simulink model "untitled1"  (R2020b)
settings: Solver=VariableStepAuto  StartTime=0.0  StopTime=10.0  RelTol=1e-3
model workspace (MAT data in the model file):
  f = -1
undefined symbols (not defined in the file or in its folder): duration, effort, index, joint_name, left_wheel_hinge, model_name, pioneer2dx, right_wheel_hinge, sampleTime, waypoints
libraries: robotgazebolib x13, simulink x4, robotcorelib x3, robotalgslib x1
settings Model: Creator=tfpeng  LastModifiedBy=tfpeng

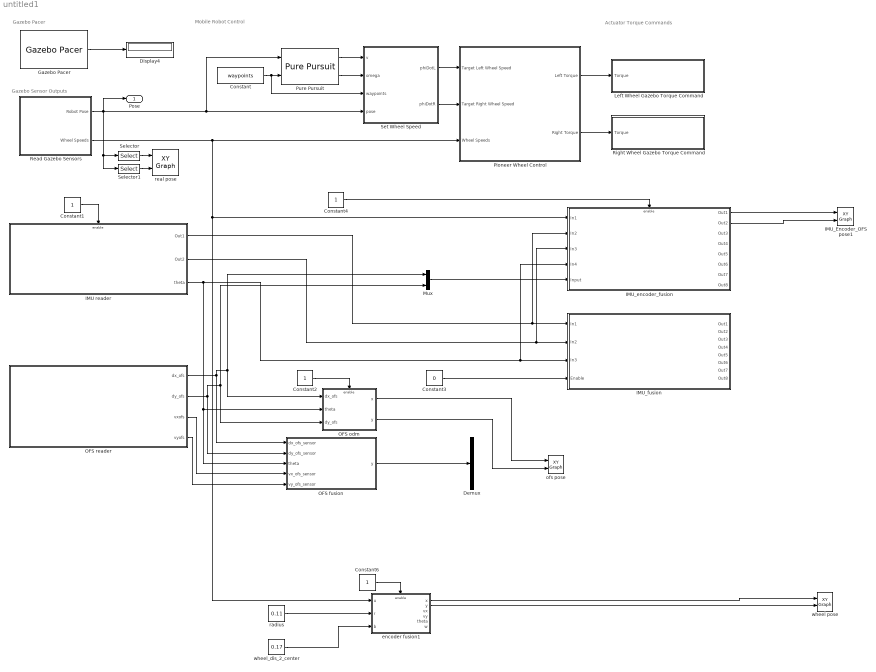
== system untitled1 ==
  note: Gazebo Pacer
  note: Actuator Torque Commands
  note: Mobile Robot Control
  note: Gazebo Sensor Outputs
  Constant : Constant  Value=waypoints
  Constant{1..2,4,6} (4 alike) : Constant
  Constant3 : Constant  Value=0
  Demux : Demux  Outputs=8
  Display4 : Display
  Gazebo Pacer : robotgazebolib/Gazebo Pacer  ResetBehavior=Reset Gazebo simulation time and scene  SampleTime=0.01
      settings: SourceProductName=Robotics System Toolbox
  IMU reader : Subsystem
  IMU_Encoder_OFS pose1 : simulink/Sinks/XY Graph  xmin=-1  xmax=4  ymin=-1  ymax=8  st=-1
  IMU_encoder_fusion : Subsystem
  IMU_fusion : Subsystem
  Left Wheel Gazebo Torque Command : Subsystem
  Mux : Mux  Inputs=2
  OFS fusion : MATLAB Function  TreatAsAtomicUnit=on
  OFS odm : Subsystem
  OFS reader : Subsystem
  Pioneer Wheel Control : Subsystem
  Pure Pursuit : robotalgslib/Pure Pursuit  DesiredLinearVelocity=1.0  MaxAngularVelocity=1.0  LookaheadDistance=1.0  TargetDirPort=off  SimulateUsing=Code generation
  Read Gazebo Sensors : Subsystem
  Right Wheel Gazebo Torque Command : Subsystem
  Selector : Selector  InputPortWidth=3  IndexOptions=Index vector (dialog)  Indices=[1]  OutputSizes=1
  Selector1 : Selector  InputPortWidth=3  IndexOptions=Index vector (dialog)  Indices=[2]  OutputSizes=1
  Set Wheel Speed : MATLAB Function  TreatAsAtomicUnit=on
  encoder fusion1 : Subsystem  TreatAsAtomicUnit=on
  ofs pose : simulink/Sinks/XY Graph  xmin=-1  xmax=4  ymin=-1  ymax=8  st=-1
  radius : Constant  Value=0.11
  real pose : simulink/Sinks/XY Graph  xmin=-1  xmax=4  ymin=-1  ymax=8  st=-1
  wheel pose : simulink/Sinks/XY Graph  xmin=-1  xmax=4  ymin=-1  ymax=8  st=-1
  wheel_dis_2_center : Constant  Value=0.17
  Pose : Outport
  wires:
  Pure Pursuit/2 -> Set Wheel Speed/2(omega)
  Constant/1 -> Set Wheel Speed/3(waypoints), Pure Pursuit/2
  Pioneer Wheel Control/2(Right Torque) -> Right Wheel Gazebo Torque Command/1(Torque)
  Pure Pursuit/1 -> Set Wheel Speed/1(v)
  Read Gazebo Sensors/1(Robot Pose) -> Selector1/1, Selector/1, Pure Pursuit/1, Set Wheel Speed/4(pose), Pose/1
  Set Wheel Speed/2(phiDotR) -> Pioneer Wheel Control/2(Target Right Wheel Speed)
  Set Wheel Speed/1(phiDotL) -> Pioneer Wheel Control/1(Target Left Wheel Speed)
  Pioneer Wheel Control/1(Left Torque) -> Left Wheel Gazebo Torque Command/1(Torque)
  Gazebo Pacer/1 -> Display4/1
  Read Gazebo Sensors/2(Wheel Speeds) -> encoder fusion1/1(u), IMU_encoder_fusion/1(In1), Pioneer Wheel Control/3(Wheel Speeds)
  radius/1 -> encoder fusion1/2(r)
  wheel_dis_2_center/1 -> encoder fusion1/3(b)
  Selector/1 -> real pose/1
  Selector1/1 -> real pose/2
  Constant4/1 -> IMU_encoder_fusion/Enable
  Constant6/1 -> encoder fusion1/Enable
  encoder fusion1/1(x) -> wheel pose/1
  encoder fusion1/2(y) -> wheel pose/2
  IMU reader/1(Out1) -> IMU_encoder_fusion/2(In2), IMU_fusion/1(In1)
  IMU reader/2(Out2) -> IMU_encoder_fusion/3(In3), IMU_fusion/2(In2)
  Constant3/1 -> IMU_fusion/4(Enable)
  Constant1/1 -> IMU reader/Enable
  IMU_encoder_fusion/1(Out1) -> IMU_Encoder_OFS pose1/1
  IMU_encoder_fusion/2(Out2) -> IMU_Encoder_OFS pose1/2
  OFS reader/1(dx_ofs) -> OFS odm/1(dx_ofs), Mux/1, OFS fusion/1(dx_ofs_sensor)
  OFS reader/2(dy_ofs) -> OFS odm/3(dy_ofs), Mux/2, OFS fusion/2(dy_ofs_sensor)
  Mux/1 -> IMU_encoder_fusion/5(Input)
  IMU reader/3(theta) -> OFS fusion/3(theta), OFS odm/2(theta), IMU_encoder_fusion/4(In4), IMU_fusion/3(In3)
  Constant2/1 -> OFS odm/Enable
  OFS reader/3(vxofs) -> OFS fusion/4(vx_ofs_sensor)
  OFS reader/4(vyofs) -> OFS fusion/5(vy_ofs_sensor)
  OFS fusion/1(y) -> Demux/1
  OFS odm/1(x) -> ofs pose/1
  OFS odm/2(y) -> ofs pose/2

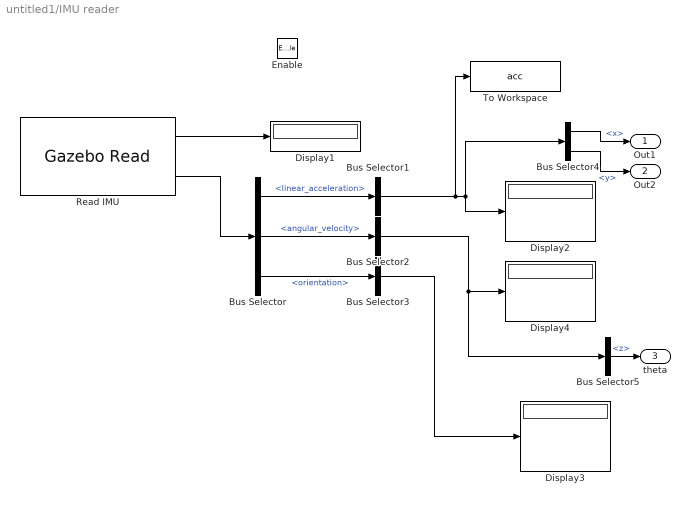
== system untitled1/IMU reader ==
  Enable : EnablePort
  Bus Selector : BusSelector  OutputSignals=linear_acceleration,angular_velocity,orientation
  Bus Selector1 : BusSelector  OutputSignals=x,y,z  OutputAsBus=on
  Bus Selector2 : BusSelector  OutputSignals=x,y,z  OutputAsBus=on
  Bus Selector3 : BusSelector  OutputSignals=w,x,y,z  OutputAsBus=on
  Bus Selector4 : BusSelector  OutputSignals=x,y
  Bus Selector5 : BusSelector  OutputSignals=z
  Display{1..4} (4 alike) : Display
      Display2 settings: Decimation=3
      Display3 settings: Decimation=3
      Display4 settings: Decimation=3
  Read IMU : robotgazebolib/Gazebo Read  topicSource=From Gazebo  topic=/gazebo/default/pioneer2dx/imu/imu/imu  messageType=gazebo_msgs/IMU  sampleTime=0.01
      settings: SourceProductName=Robotics System Toolbox
  To Workspace : ToWorkspace  VariableName=acc  SaveFormat=Timeseries  SampleTime=-1
      settings: Decimation=3
  Out1 : Outport
  Out2 : Outport  Port=2
  theta : Outport  Port=3
  wires:
  Bus Selector2/1 -> Bus Selector5/1, Display4/1
  Read IMU/1 -> Display1/1
  Read IMU/2 -> Bus Selector/1
  Bus Selector3/1 -> Display3/1
  Bus Selector/3 -> Bus Selector3/1  "<orientation>"
  Bus Selector/1 -> Bus Selector1/1  "<linear_acceleration>"
  Bus Selector1/1 -> To Workspace/1, Display2/1, Bus Selector4/1
  Bus Selector/2 -> Bus Selector2/1  "<angular_velocity>"
  Bus Selector4/1 -> Out1/1  "<x>"
  Bus Selector4/2 -> Out2/1  "<y>"
  Bus Selector5/1 -> theta/1  "<z>"

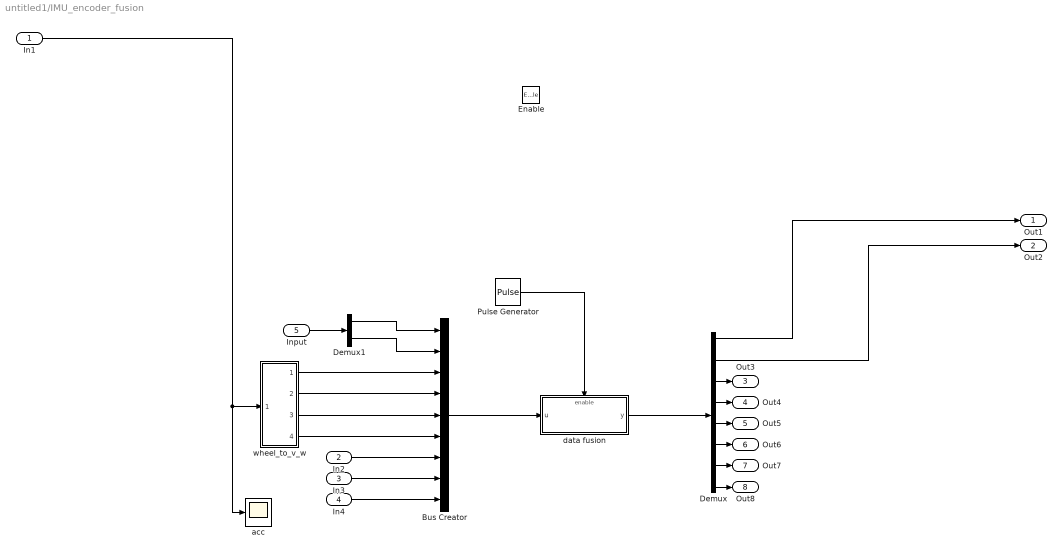
== system untitled1/IMU_encoder_fusion ==
  In1 : Inport
  In2 : Inport  Port=2
  In3 : Inport  Port=3
  In4 : Inport  Port=4
  Input : Inport  Port=5
  Enable : EnablePort
  Bus Creator : BusCreator  Inputs=9
  Demux : Demux  Outputs=8
  Demux1 : Demux  Outputs=2
  Pulse Generator : DiscretePulseGenerator  PulseType=Time based  Period=0.01  PulseWidth=50
  acc : Scope
  data fusion : Subsystem  TreatAsAtomicUnit=on
  wheel_to_v_w : Subsystem
  Out1 : Outport
  Out2 : Outport  Port=2
  Out3 : Outport  Port=3
  Out4 : Outport  Port=4
  Out5 : Outport  Port=5
  Out6 : Outport  Port=6
  Out7 : Outport  Port=7
  Out8 : Outport  Port=8
  wires:
  wheel_to_v_w/1(Out1) -> Bus Creator/3
  Demux/7 -> Out7/1
  Demux/8 -> Out8/1
  Pulse Generator/1 -> data fusion/Enable
  Demux/2 -> Out2/1
  In2/1 -> Bus Creator/7
  Demux/3 -> Out3/1
  In4/1 -> Bus Creator/9
  In1/1 -> acc/1, wheel_to_v_w/1(In1)
  In3/1 -> Bus Creator/8
  data fusion/1(y) -> Demux/1
  Demux/4 -> Out4/1
  Demux/1 -> Out1/1
  Demux/5 -> Out5/1
  Bus Creator/1 -> data fusion/1(u)
  Demux/6 -> Out6/1
  wheel_to_v_w/3(Out4) -> Bus Creator/5
  wheel_to_v_w/2(Out3) -> Bus Creator/4
  wheel_to_v_w/4(Out2) -> Bus Creator/6
  Input/1 -> Demux1/1
  Demux1/1 -> Bus Creator/1
  Demux1/2 -> Bus Creator/2

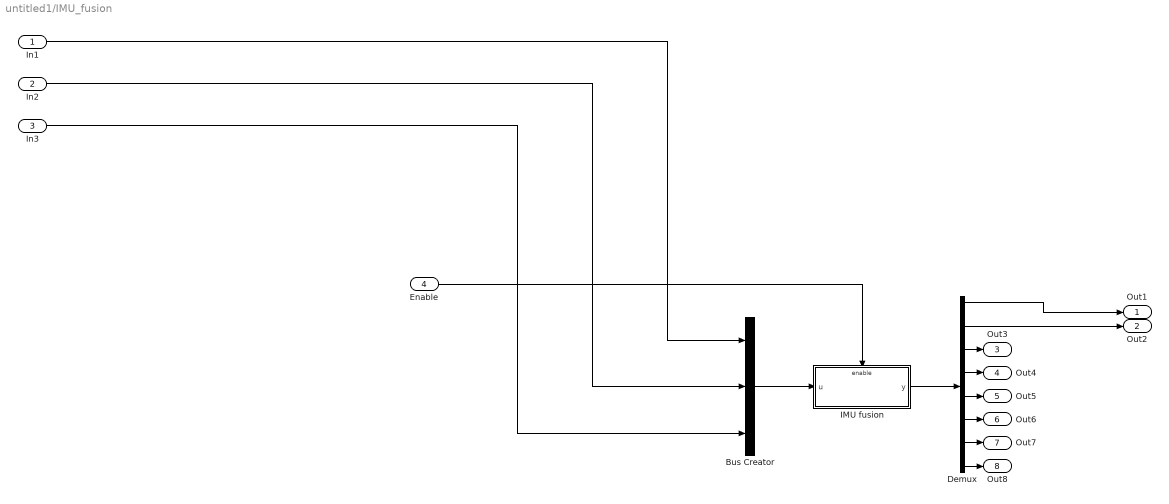
== system untitled1/IMU_fusion ==
  In1 : Inport
  In2 : Inport  Port=2
  In3 : Inport  Port=3
  Enable : Inport  Port=4
  Bus Creator : BusCreator  Inputs=3
  Demux : Demux  Outputs=8
  IMU fusion : Subsystem  TreatAsAtomicUnit=on
  Out1 : Outport
  Out2 : Outport  Port=2
  Out3 : Outport  Port=3
  Out4 : Outport  Port=4
  Out5 : Outport  Port=5
  Out6 : Outport  Port=6
  Out7 : Outport  Port=7
  Out8 : Outport  Port=8
  wires:
  Demux/3 -> Out3/1
  Enable/1 -> IMU fusion/Enable
  Demux/5 -> Out5/1
  Bus Creator/1 -> IMU fusion/1(u)
  In3/1 -> Bus Creator/3
  Demux/4 -> Out4/1
  IMU fusion/1(y) -> Demux/1
  Demux/6 -> Out6/1
  In2/1 -> Bus Creator/2
  In1/1 -> Bus Creator/1
  Demux/7 -> Out7/1
  Demux/2 -> Out2/1
  Demux/8 -> Out8/1
  Demux/1 -> Out1/1

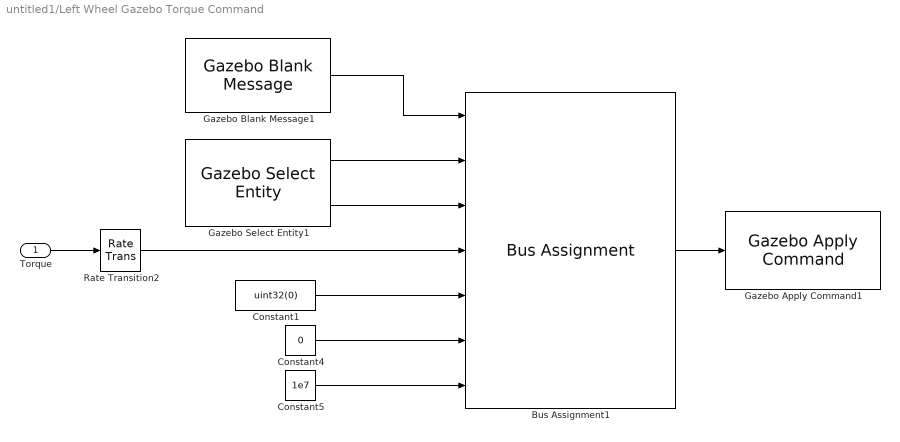
== system untitled1/Left Wheel Gazebo Torque Command ==
  Torque : Inport
  Bus Assignment1 : BusAssignment  AssignedSignals=model_name,joint_name,effort,index,duration.seconds,duration.nano_seconds
  Constant1 : Constant  Value=uint32(0)
  Constant4 : Constant  Value=0
  Constant5 : Constant  Value=1e7
  Gazebo Apply Command1 : robotgazebolib/Gazebo Apply Command  cmdType=ApplyJointTorque  sampleTime=0.01
      settings: SourceProductName=Robotics System Toolbox
  Gazebo Blank Message1 : robotgazebolib/Gazebo Blank Message  msgType=ApplyJointTorque  sampleTime=0.01  busName='Gazebo_SL_Bus_gazebo_msgs_ApplyJointTorque'
      settings: SourceProductName=Robotics System Toolbox
  Gazebo Select Entity1 : robotgazebolib/Gazebo Select Entity  modelElemName=pioneer2dx/left_wheel_hinge  outputArraySize=128  OutputLabel=Joint  SelectType=Joint
      settings: SourceProductName=Robotics System Toolbox
  Rate Transition2 : RateTransition
  wires:
  Bus Assignment1/1 -> Gazebo Apply Command1/1
  Constant5/1 -> Bus Assignment1/7
  Gazebo Blank Message1/1 -> Bus Assignment1/1
  Gazebo Select Entity1/2 -> Bus Assignment1/3
  Gazebo Select Entity1/1 -> Bus Assignment1/2
  Torque/1 -> Rate Transition2/1
  Constant4/1 -> Bus Assignment1/6
  Rate Transition2/1 -> Bus Assignment1/4
  Constant1/1 -> Bus Assignment1/5

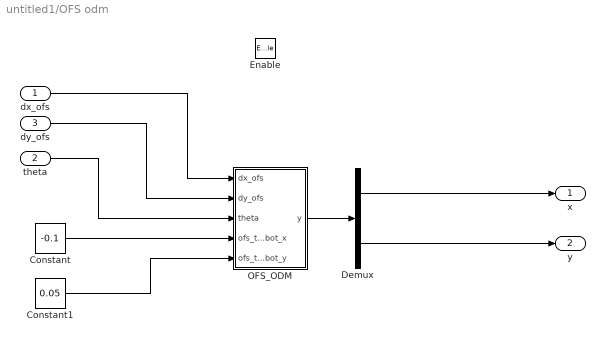
== system untitled1/OFS odm ==
  dx_ofs : Inport
  theta : Inport  Port=2
  dy_ofs : Inport  Port=3
  Enable : EnablePort
  Constant : Constant  Value=-0.1
  Constant1 : Constant  Value=0.05
  Demux : Demux  Outputs=2
  OFS_ODM : MATLAB Function  TreatAsAtomicUnit=on
  x : Outport
  y : Outport  Port=2
  wires:
  Demux/2 -> y/1
  Demux/1 -> x/1
  theta/1 -> OFS_ODM/3(theta)
  dx_ofs/1 -> OFS_ODM/1(dx_ofs)
  OFS_ODM/1(y) -> Demux/1
  dy_ofs/1 -> OFS_ODM/2(dy_ofs)
  Constant/1 -> OFS_ODM/4(ofs_to_robot_x)
  Constant1/1 -> OFS_ODM/5(ofs_to_robot_y)

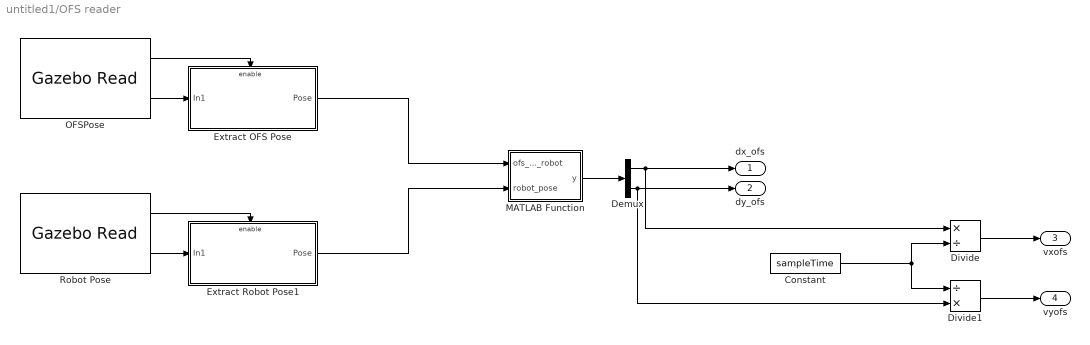
== system untitled1/OFS reader ==
  Constant : Constant  Value=sampleTime
  Demux : Demux  Outputs=2
  Divide : Product  Inputs=*/
  Divide1 : Product  Inputs=/*
  Extract OFS Pose : Subsystem
  Extract Robot Pose1 : Subsystem
  MATLAB Function : MATLAB Function  TreatAsAtomicUnit=on
  OFSPose : robotgazebolib/Gazebo Read  topicSource=From Gazebo  topic=/gazebo/ground_truth/link_state/pioneer2dx/ofs  messageType=gazebo_msgs/LinkState  sampleTime=0.01
      settings: SourceProductName=Robotics System Toolbox
  Robot Pose : robotgazebolib/Gazebo Read  topicSource=From Gazebo  topic=/gazebo/ground_truth/world_pose/pioneer2dx/chassis  messageType=gazebo_msgs/Pose  sampleTime=0.01
      settings: SourceProductName=Robotics System Toolbox
  dx_ofs : Outport
  dy_ofs : Outport  Port=2
  vxofs : Outport  Port=3
  vyofs : Outport  Port=4
  wires:
  Extract Robot Pose1/1(Pose) -> MATLAB Function/2(robot_pose)
  Extract OFS Pose/1(Pose) -> MATLAB Function/1(ofs_pose_robot)
  MATLAB Function/1(y) -> Demux/1
  Robot Pose/1 -> Extract Robot Pose1/Enable
  OFSPose/1 -> Extract OFS Pose/Enable
  Robot Pose/2 -> Extract Robot Pose1/1(In1)
  OFSPose/2 -> Extract OFS Pose/1(In1)
  Demux/1 -> dx_ofs/1, Divide/1
  Demux/2 -> Divide1/2, dy_ofs/1
  Constant/1 -> Divide/2, Divide1/1
  Divide/1 -> vxofs/1
  Divide1/1 -> vyofs/1

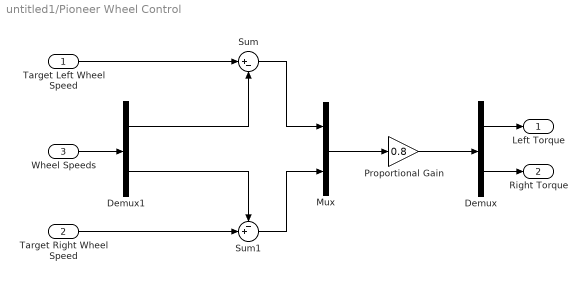
== system untitled1/Pioneer Wheel Control ==
  Target Left Wheel Speed : Inport
  Target Right Wheel Speed : Inport  Port=2
  Wheel Speeds : Inport  Port=3
  Demux : Demux  Outputs=2
  Demux1 : Demux  Outputs=2
  Mux : Mux  Inputs=2
  Proportional Gain : Gain  Gain=0.8
  Sum : Sum  Inputs=|+-
  Sum1 : Sum  Inputs=-+|
  Left Torque : Outport
  Right Torque : Outport  Port=2
  wires:
  Sum1/1 -> Mux/2
  Target Left Wheel Speed/1 -> Sum/1
  Sum/1 -> Mux/1
  Mux/1 -> Proportional Gain/1
  Proportional Gain/1 -> Demux/1
  Demux/1 -> Left Torque/1
  Demux/2 -> Right Torque/1
  Wheel Speeds/1 -> Demux1/1
  Demux1/1 -> Sum/2
  Target Right Wheel Speed/1 -> Sum1/2
  Demux1/2 -> Sum1/1

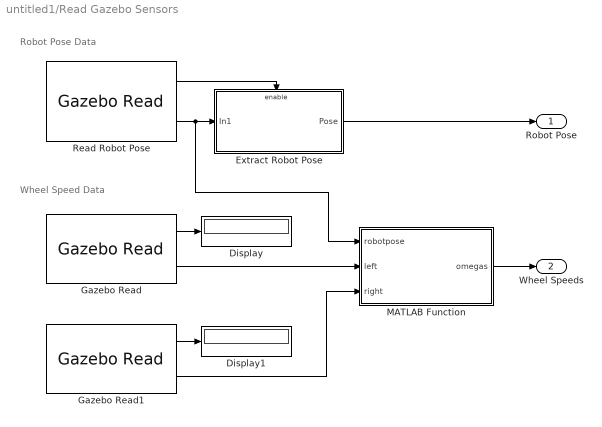
== system untitled1/Read Gazebo Sensors ==
  note: Robot Pose Data
  note: Wheel Speed Data
  Display : Display
  Display1 : Display
  Extract Robot Pose : Subsystem
  Gazebo Read : robotgazebolib/Gazebo Read  topicSource=From Gazebo  topic=/gazebo/ground_truth/world_pose/pioneer2dx/left_wheel  messageType=gazebo_msgs/Pose  sampleTime=0.01
      settings: SourceProductName=Robotics System Toolbox
  Gazebo Read1 : robotgazebolib/Gazebo Read  topicSource=From Gazebo  topic=/gazebo/ground_truth/world_pose/pioneer2dx/right_wheel  messageType=gazebo_msgs/Pose  sampleTime=0.01
      settings: SourceProductName=Robotics System Toolbox
  MATLAB Function : MATLAB Function  TreatAsAtomicUnit=on
  Read Robot Pose : robotgazebolib/Gazebo Read  topicSource=From Gazebo  topic=/gazebo/ground_truth/world_pose/pioneer2dx/chassis  messageType=gazebo_msgs/Pose  sampleTime=0.01
      settings: SourceProductName=Robotics System Toolbox
  Robot Pose : Outport
  Wheel Speeds : Outport  Port=2
  wires:
  Read Robot Pose/2 -> MATLAB Function/1(robotpose), Extract Robot Pose/1(In1)
  Extract Robot Pose/1(Pose) -> Robot Pose/1
  Read Robot Pose/1 -> Extract Robot Pose/Enable
  Gazebo Read/1 -> Display/1
  Gazebo Read1/1 -> Display1/1
  MATLAB Function/1(omegas) -> Wheel Speeds/1
  Gazebo Read/2 -> MATLAB Function/2(left)
  Gazebo Read1/2 -> MATLAB Function/3(right)

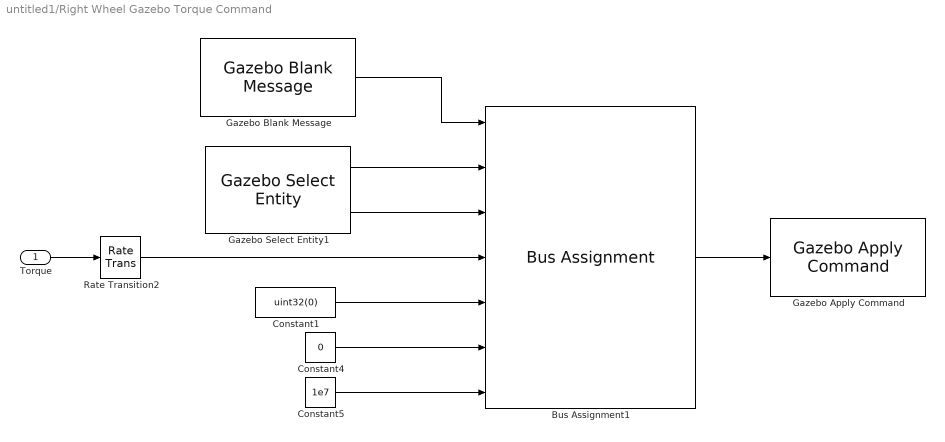
== system untitled1/Right Wheel Gazebo Torque Command ==
  Torque : Inport
  Bus Assignment1 : BusAssignment  AssignedSignals=model_name,joint_name,effort,index,duration.seconds,duration.nano_seconds
  Constant1 : Constant  Value=uint32(0)
  Constant4 : Constant  Value=0
  Constant5 : Constant  Value=1e7
  Gazebo Apply Command : robotgazebolib/Gazebo Apply Command  cmdType=ApplyJointTorque  sampleTime=0.01
      settings: SourceProductName=Robotics System Toolbox
  Gazebo Blank Message : robotgazebolib/Gazebo Blank Message  msgType=ApplyJointTorque  sampleTime=0.01  busName='Gazebo_SL_Bus_gazebo_msgs_ApplyJointTorque'
      settings: SourceProductName=Robotics System Toolbox
  Gazebo Select Entity1 : robotgazebolib/Gazebo Select Entity  modelElemName=pioneer2dx/right_wheel_hinge  outputArraySize=128  OutputLabel=Joint  SelectType=Joint
      settings: SourceProductName=Robotics System Toolbox
  Rate Transition2 : RateTransition
  wires:
  Constant1/1 -> Bus Assignment1/5
  Rate Transition2/1 -> Bus Assignment1/4
  Constant4/1 -> Bus Assignment1/6
  Torque/1 -> Rate Transition2/1
  Gazebo Select Entity1/1 -> Bus Assignment1/2
  Gazebo Select Entity1/2 -> Bus Assignment1/3
  Gazebo Blank Message/1 -> Bus Assignment1/1
  Constant5/1 -> Bus Assignment1/7
  Bus Assignment1/1 -> Gazebo Apply Command/1

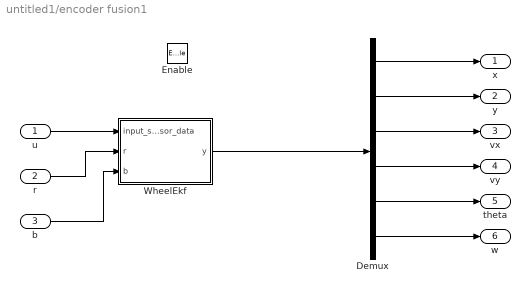
== system untitled1/encoder fusion1 ==
  u : Inport
  r : Inport  Port=2
  b : Inport  Port=3
  Enable : EnablePort
  Demux : Demux  Outputs=6
  WheelEkf : MATLAB Function  TreatAsAtomicUnit=on
  x : Outport
  y : Outport  Port=2
  vx : Outport  Port=3
  vy : Outport  Port=4
  theta : Outport  Port=5
  w : Outport  Port=6
  wires:
  u/1 -> WheelEkf/1(input_sensor_data)
  WheelEkf/1(y) -> Demux/1
  r/1 -> WheelEkf/2(r)
  b/1 -> WheelEkf/3(b)
  Demux/1 -> x/1
  Demux/2 -> y/1
  Demux/3 -> vx/1
  Demux/4 -> vy/1
  Demux/5 -> theta/1
  Demux/6 -> w/1

== system untitled1/IMU_encoder_fusion/data fusion ==
  u : Inport
  Enable : EnablePort
  PoseEstimationEkf : MATLAB Function  TreatAsAtomicUnit=on
  y : Outport
  wires:
  u/1 -> PoseEstimationEkf/1(input_sensor_data)
  PoseEstimationEkf/1(y) -> y/1

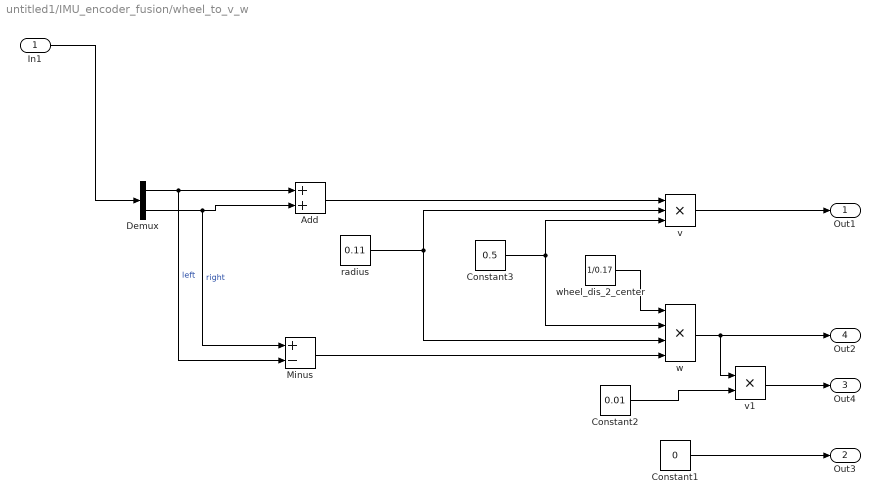
== system untitled1/IMU_encoder_fusion/wheel_to_v_w ==
  In1 : Inport
  Add : Sum
  Constant1 : Constant  Value=0
  Constant2 : Constant  Value=0.01
  Constant3 : Constant  Value=0.5
  Demux : Demux  Outputs=2
  Minus : Sum  Inputs=+-
  radius : Constant  Value=0.11
  v : Product  Inputs=3
  v1 : Product
  w : Product  Inputs=4
  wheel_dis_2_center : Constant  Value=1/0.17
  Out1 : Outport
  Out3 : Outport  Port=2
  Out4 : Outport  Port=3
  Out2 : Outport  Port=4
  wires:
  Minus/1 -> w/4
  w/1 -> v1/1, Out2/1
  In1/1 -> Demux/1
  Add/1 -> v/1
  wheel_dis_2_center/1 -> w/1
  v/1 -> Out1/1
  radius/1 -> w/3, v/2
  Demux/2 -> Minus/1, Add/2  "right"
  Demux/1 -> Minus/2, Add/1  "left"
  Constant3/1 -> w/2, v/3
  Constant1/1 -> Out3/1
  Constant2/1 -> v1/2
  v1/1 -> Out4/1

== system untitled1/IMU_fusion/IMU fusion ==
  u : Inport
  Enable : EnablePort
  PoseEstimationEkf : MATLAB Function  TreatAsAtomicUnit=on
  y : Outport
  wires:
  u/1 -> PoseEstimationEkf/1(input_sensor_data)
  PoseEstimationEkf/1(y) -> y/1

== system untitled1/OFS reader/Extract OFS Pose ==
  note: Generate a pose vector (x, y, theta) from X, Y, and quaternion data
  In1 : Inport
  Enable : EnablePort
  Bus Selector1 : BusSelector  OutputSignals=relative_pose.position.x,relative_pose.position.y,relative_pose.orientation.w,relative_pose.orientation.x,relative_pose.orientation.y,relative_pose.orientation.z
  Coordinate Transformation Conversion : robotcorelib/Coordinate Transformation Conversion  InputRepresentation=Quaternion  InputEulerSequence=ZYX  ShowTrVecInputPort=on  OutputRepresentation=Euler Angles  OutputEulerSequence=ZYX  ShowTrVecOutputPort=on  SimulateUsing=Interpreted execution
  Mux2 : Mux  Inputs=3
  Selector2 : Selector  InputPortWidth=3  IndexOptions=Index vector (dialog)  Indices=1  OutputSizes=1
  Vector Concatenate : Concatenate  NumInputs=4
  Pose : Outport  VectorParamsAs1DForOutWhenUnconnected=off
  wires:
  Vector Concatenate/1 -> Coordinate Transformation Conversion/1
  Coordinate Transformation Conversion/1 -> Selector2/1
  Selector2/1 -> Mux2/3
  Mux2/1 -> Pose/1
  Bus Selector1/6 -> Vector Concatenate/4  "<z>"
  Bus Selector1/1 -> Mux2/1  "<x>"
  Bus Selector1/4 -> Vector Concatenate/2  "<x>"
  Bus Selector1/2 -> Mux2/2  "<y>"
  Bus Selector1/3 -> Vector Concatenate/1  "<w>"
  Bus Selector1/5 -> Vector Concatenate/3  "<y>"
  In1/1 -> Bus Selector1/1

== system untitled1/OFS reader/Extract Robot Pose1 ==
  note: Generate a pose vector (x, y, theta) from X, Y, and quaternion data
  In1 : Inport
  Enable : EnablePort
  Bus Selector1 : BusSelector  OutputSignals=position.x,position.y,orientation.w,orientation.x,orientation.y,orientation.z
  Coordinate Transformation Conversion : robotcorelib/Coordinate Transformation Conversion  InputRepresentation=Quaternion  InputEulerSequence=ZYX  ShowTrVecInputPort=on  OutputRepresentation=Euler Angles  OutputEulerSequence=ZYX  ShowTrVecOutputPort=on  SimulateUsing=Interpreted execution
  Mux1 : Mux  Inputs=2
  Mux2 : Mux  Inputs=2
  Selector2 : Selector  InputPortWidth=3  IndexOptions=Index vector (dialog)  Indices=1  OutputSizes=1
  Vector Concatenate : Concatenate  NumInputs=4
  Pose : Outport  VectorParamsAs1DForOutWhenUnconnected=off
  wires:
  Vector Concatenate/1 -> Coordinate Transformation Conversion/1
  Coordinate Transformation Conversion/1 -> Selector2/1
  Mux1/1 -> Mux2/1
  Selector2/1 -> Mux2/2
  Mux2/1 -> Pose/1
  Bus Selector1/6 -> Vector Concatenate/4  "<z>"
  Bus Selector1/1 -> Mux1/1  "<x>"
  Bus Selector1/4 -> Vector Concatenate/2  "<x>"
  Bus Selector1/2 -> Mux1/2  "<y>"
  Bus Selector1/3 -> Vector Concatenate/1  "<w>"
  Bus Selector1/5 -> Vector Concatenate/3  "<y>"
  In1/1 -> Bus Selector1/1

== system untitled1/Read Gazebo Sensors/Extract Robot Pose ==
  note: Generate a pose vector (x, y, theta) from X, Y, and quaternion data
  In1 : Inport
  Enable : EnablePort
  Bus Selector1 : BusSelector  OutputSignals=position.x,position.y,orientation.w,orientation.x,orientation.y,orientation.z
  Coordinate Transformation Conversion : robotcorelib/Coordinate Transformation Conversion  InputRepresentation=Quaternion  InputEulerSequence=ZYX  ShowTrVecInputPort=on  OutputRepresentation=Euler Angles  OutputEulerSequence=ZYX  ShowTrVecOutputPort=on  SimulateUsing=Interpreted execution
  Mux1 : Mux  Inputs=2
  Mux2 : Mux  Inputs=2
  Selector2 : Selector  InputPortWidth=3  IndexOptions=Index vector (dialog)  Indices=1  OutputSizes=1
  Vector Concatenate : Concatenate  NumInputs=4
  Pose : Outport  VectorParamsAs1DForOutWhenUnconnected=off
  wires:
  Vector Concatenate/1 -> Coordinate Transformation Conversion/1
  Coordinate Transformation Conversion/1 -> Selector2/1
  Mux1/1 -> Mux2/1
  Selector2/1 -> Mux2/2
  Mux2/1 -> Pose/1
  Bus Selector1/6 -> Vector Concatenate/4  "<z>"
  Bus Selector1/1 -> Mux1/1  "<x>"
  Bus Selector1/4 -> Vector Concatenate/2  "<x>"
  Bus Selector1/2 -> Mux1/2  "<y>"
  Bus Selector1/3 -> Vector Concatenate/1  "<w>"
  Bus Selector1/5 -> Vector Concatenate/3  "<y>"
  In1/1 -> Bus Selector1/1

== matlab function untitled1/Read Gazebo Sensors/MATLAB Function ==
  data: robotpose input; omegas output; left input; right input
function omegas = computeWheelVelocities(robotpose, left, right)
%computeWheelVelocities computes wheel velocity based on rate of change of
%the yaw angle of the wheel relative to its original mount on the robot
%body

persistent initAngles
if isempty(initAngles)
    initAngles = zeros(2,1);
end
sampleTime = 0.01;

% compute rotation between wheel original mount on the robot body and world
% frame
robotRtom = quat2rotm([robotpose.orientation.w, robotpose.orientation.x, robotpose.orientation.y, robotpose.orientation.z]);
originalWheelMount = robotRtom*eul2rotm([pi/2 pi/2 0]);

% get rotation between wheel and the world frame
leftRtom = quat2rotm([left.orientation.w, left.orientation.x, left.orientation.y, left.orientation.z]);
rightRtom = quat2rotm([right.orientation.w, right.orientation.x, right.orientation.y, right.orientation.z]);

% compute relative rotation between wheel and its original mount
leftRotation = rotm2eul(originalWheelMount'*leftRtom);
rightRotation = rotm2eul(originalWheelMount'*rightRtom);

% compute angluar velocity using the angle difference between the current
% angle pose and the the angle pose in last time step
angles = [leftRotation(1); rightRotation(1)];
omegas = angdiff(initAngles, angles)/sampleTime;
initAngles = angles;

== matlab function untitled1/Set Wheel Speed ==
  data: v input; omega input; waypoints input; pose input; phiDotL output; phiDotR output
function [phiDotL, phiDotR] = wheelSpeed(v, omega, waypoints, pose)

% Path constants
stopThreshold = 0.1;
slowThreshold = 0.3;

% Robot constants
trackWidth = 0.381;
wheelRadius = 0.195/2;

% Slow the robot down when it's near the threshold
distanceToEndpoint = norm(waypoints(end, :) - pose(1:2)');
if (distanceToEndpoint < slowThreshold)
    v = distanceToEndpoint/slowThreshold*v;
    
    % Stop the robot if it's inside the target threshold
    if distanceToEndpoint < stopThreshold
        v = 0;
    end
end

% Convert velocity and heading angular velocity to wheel speeds
phiDotL = (v - trackWidth/2*omega)/wheelRadius;
phiDotR = (v + trackWidth/2*omega)/wheelRadius;

end

== matlab function untitled1/IMU_encoder_fusion/data fusion/PoseEstimationEkf ==
  data: input_sensor_data input; y output
function y = PoseEstimationEkf(input_sensor_data)
persistent state_variable_current state_variable_last P Q counter;
if isempty(state_variable_current)
        state_variable_current=zeros(8,1);%[xt,yt,theta_t,vxt,vyt,wt,axt,ayt]
        state_variable_last=zeros(8,1);
        Q=diag([0.1, 0.1, 0.1,0.1, 0.1, 0.1, 0.1, 0.1]);
        P=Q;
        counter=0;
end

%%    predict
dt=0.01;
A=[[1, 0, 0, dt, 0, 0, 0.5*dt^2, 0]
  [0, 1, 0, 0, dt, 0, 0, 0.5*dt^2]
  [0, 0, 1, 0, 0, dt, 0, 0]
  [0, 0, 0, 1, 0, 0, dt, 0]
  [0, 0, 0, 0, 1, 0, 0, dt]
  [0, 0, 0, 0, 0, 1, 0, 0]
  [0, 0, 0, 0, 0, 0, 1, 0]
  [0, 0, 0, 0, 0, 0, 0, 1]];
state_variable_current=A*state_variable_current;
P=A*P*A'+Q;

%%    update
theta=state_variable_current(3);
theta_last=state_variable_last(3);
vx=state_variable_current(4);
vy=state_variable_current(5);
ax=state_variable_current(7);
ay=state_variable_current(8);
dx=state_variable_current(1)-state_variable_last(1);
dy=state_variable_current(2)-state_variable_last(2);
w=state_variable_current(6);
dtheta=theta-theta_last;
v=vx*cos(theta)+vy*sin(theta);
vr=vx*sin(theta)-vy*cos(theta);
dd=sqrt(dx^2+dy^2);
ax_imu=ax*cos(theta)+ay*sin(theta);
ay_imu=-ax*sin(theta)+ay*cos(theta);
dx_ofs=dd*cos(dtheta/2);
dy_ofs=dd*sin(dtheta/2);
%% all sensor data fusion  --not debug
H=[[cos(0.5*dtheta)*cos(theta_last+0.5*dtheta), cos(0.5*dtheta)*sin(theta_last+0.5*dtheta), -0.5*dd*sin(0.5*dtheta), 0, 0, 0, 0, 0]
   [sin(0.5*dtheta)*cos(theta_last+0.5*dtheta), sin(0.5*dtheta)*sin(theta_last+0.5*dtheta), 0.5*dd*cos(0.5*dtheta), 0, 0, 0, 0, 0]
  [0, 0, -vx*sin(theta)+vy*cos(theta), cos(theta), sin(theta), 0, 0, 0]
  [0, 0, vx*cos(theta)+vy*sin(theta), sin(theta), -cos(theta), 0, 0, 0]
  [0, 0, 1, 0, 0, 0, 0, 0]
  [0, 0, 0, 0, 0, 1, 0, 0]
  [0, 0, -ax*sin(theta)+ay*cos(theta), 0, 0, 0, cos(theta), sin(theta)]
  [0, 0, -ax*cos(theta)-ay*sin(theta), 0, 0, 0, -sin(theta), cos(theta)]
  [0, 0, 0, 0, 0, 1, 0, 0]
  [0, 0, 1, 0, 0, 0, 0, 0]];
Z=[dx_ofs,dy_ofs,v,vr,dtheta, w,ax_imu, ay_imu,w,dtheta]';
R = diag([0.001,0.001,0.001,0.001,0.001,0.001,0.0002,0.0002,0.0002,0.0002]);
encoder_input_sensor_data=input_sensor_data(3:6);
imu_input_sensor_data=[input_sensor_data(7:9);input_sensor_data(9)*dt];
ofs_input_sensor_data=input_sensor_data(1:2);

temp_input_data=[ofs_input_sensor_data;encoder_input_sensor_data;imu_input_sensor_data];
error=temp_input_data-Z;
%% just wheel encoder fusion  --debug ok
% H=[[0, 0, -vx*sin(theta)+vy*cos(theta), cos(theta), sin(theta), 0, 0, 0]
%   [0, 0, vx*cos(theta)+vy*sin(theta), sin(theta), -cos(theta), 0, 0, 0]
%   [0, 0, 1, 0, 0, 0, 0, 0]
%   [0, 0, 0, 0, 0, 1, 0, 0]];
% Z=[v,vr,dtheta, w]';
% R = diag([0.001, 0.001,0.001,0.001]);
% temp_input_sensor_data=input_sensor_data(3:6);
% error=temp_input_sensor_data-Z;

%% just IMU fusion    --debug ok
% H=[[0, 0, -ax*sin(theta)+ay*cos(theta), 0, 0, 0, cos(theta), sin(theta)]
%   [0, 0, -ax*cos(theta)-ay*sin(theta), 0, 0, 0, -sin(theta), cos(theta)]
%   [0, 0, 0, 0, 0, 1, 0, 0]
%   [0, 0, 1, 0, 0, 0, 0, 0]];
% Z=[ax_imu, ay_imu,w,dtheta]';
% R = diag([0.001,0.001,0.001,0.001]);
% %[ax_imu,ay_imu,w]
% input_sensor_data=[input_sensor_data(7:9);input_sensor_data(9)*dt];
% error=input_sensor_data-Z;

%%  IMU wheel encoder   
% H=[[0, 0, -vx*sin(theta)+vy*cos(theta), cos(theta), sin(theta), 0, 0, 0]
%   [0, 0, vx*cos(theta)+vy*sin(theta), sin(theta), -cos(theta), 0, 0, 0]
%   [0, 0, 1, 0, 0, 0, 0, 0]
%   [0, 0, 0, 0, 0, 1, 0, 0]
%   [0, 0, -ax*sin(theta)+ay*cos(theta), 0, 0, 0, cos(theta), sin(theta)]
%   [0, 0, -ax*cos(theta)-ay*sin(theta), 0, 0, 0, -sin(theta), cos(theta)]
%   [0, 0, 0, 0, 0, 1, 0, 0]
%   [0, 0, 1, 0, 0, 0, 0, 0]];
% Z=[v,vr,dtheta, w,ax_imu, ay_imu,w,dtheta]';
% R = diag([0.001,0.001,0.001,0.001,0.0002,0.0002,0.0002,0.0002]);
% encoder_input_sensor_data=input_sensor_data(3:6);
% imu_input_sensor_data=[input_sensor_data(7:9);input_sensor_data(9)*dt];
% temp_input_data=[encoder_input_sensor_data;imu_input_sensor_data];
% error=temp_input_data-Z;

%% correct update
temp_p=H*P*H'+R;
kalman_gain=(P*H')/(temp_p);
correct_value=kalman_gain*error;
state_variable_current=state_variable_current+correct_value;
P=P-kalman_gain*H*P;
state_variable_last=state_variable_current;
counter=counter+1;
y = state_variable_current;

== matlab function untitled1/encoder fusion1/WheelEkf ==
  data: input_sensor_data input; y output; r input; b input
function y = WheelEkf(input_sensor_data,r,b)
persistent state_variable_current state_variable_last P Q count P_array K_array H_array input_sensor_data_extant;
if isempty(state_variable_current)
        state_variable_current=zeros(6,1);%[x,y,vx,vy,theta,w]
        state_variable_last=zeros(6,1);
        input_sensor_data_extant=zeros(4,1);
        Q=diag([0.01, 0.01, 0.01, 0.01, 0.01, 0.01]);
        P=diag([0.0001, 0.0001, 0.0001, 0.0001, 0.0001, 0.0001]);
%         Q(1,3)=0.1;
%         Q(2,4)=0.1;
%         Q(5,6)=0.1;
        count=1;
        P_array=zeros(6,6,500);
        P_array(:,:,1)=P;
        K_array=zeros(6,2,500);
        H_array=zeros(2,6,500);
end
persistent time_ms;
if isempty(time_ms)
    time_ms=tic;
    y=state_variable_current;
    return;
end
%%    predict
dt=0.01;
v_input=(input_sensor_data(1)+input_sensor_data(2))*r/2;
w_input=(input_sensor_data(2)-input_sensor_data(1))*r/2/b;
d_input=v_input*dt;
dtheta_input=w_input*dt;

A=[[1, 0, dt, 0, 0, 0]
  [0, 1, 0, dt, 0 , 0]
  [0, 0, 1, 0, 0, 0]
  [0, 0, 0, 1, 0, 0]
  [0, 0, 0, 0, 1, dt]
  [0, 0, 0, 0, 0, 1]
  ];
state_variable_current=A*state_variable_current;
P=A*P*A'+Q;

%%    update
dtheta = state_variable_current(5)-state_variable_last(5);
theta=state_variable_current(5);
theta_last=state_variable_last(5);
w=state_variable_current(6);
%% 
% v=sqrt((state_variable_current(3))^2+(state_variable_current(4))^2);
% H=[[0,0,cos(theta_last+dtheta*0.5),sin(theta_last+dtheta*0.5),0,-b]
%     [0,0,cos(theta_last+dtheta*0.5),sin(theta_last+dtheta*0.5),0,b]]/r;
% H_array(:,:,count)=H;
% Z=([v-w*b,v+w*b]/r)';%[left,right]
% R = diag([0.00001, 0.00001]);
% error=input_sensor_data-Z;
%%  
% dd=sqrt((state_variable_current(1)-state_variable_last(1))^2+(state_variable_current(2)-state_variable_last(2))^2);
% v=w*sin(dtheta/2)*dd/2;
% H=[[w*cos(theta_last+dtheta/2)*sin(dtheta/2)*0.5,w*sin(theta_last+dtheta/2)*sin(dtheta/2)*0.5,0,0,w*dd*cos(dtheta/2)*0.25,b+0.5*dd*sin(dtheta/2)]
%     [w*cos(theta_last+dtheta/2)*sin(dtheta/2)*0.5,w*sin(theta_last+dtheta/2)*sin(dtheta/2)*0.5,0,0,w*dd*cos(dtheta/2)*0.25,-b+0.5*dd*sin(dtheta/2)]]/r;
% H_array(:,:,count)=H;
% Z=([v-w*b,v+w*b]/r)';%[left,right]
% R = diag([0.00001, 0.00001]);
% error=input_sensor_data-Z;
%%
% vx=state_variable_current(3);
% vy=state_variable_current(4);
% v=vx*cos(theta)+vy*sin(theta);
% H=[[0,0,cos(theta),sin(theta),-vx*sin(theta)+vy*cos(theta),b]
%     [0,0,cos(theta),sin(theta),-vx*sin(theta)+vy*cos(theta),-b]]/r;
% H_array(:,:,count)=H;
% Z=([v-w*b,v+w*b]/r)';%[left,right]
% R = diag([0.00001, 0.00001]);
% error=input_sensor_data-Z;
%% this model is work
vr_input=0;
input_sensor_data_extant=[v_input,vr_input,dtheta_input,w_input]';
vx=state_variable_current(3);
vy=state_variable_current(4);
v=vx*cos(theta)+vy*sin(theta);
vr=vx*sin(theta)-vy*cos(theta);

H=[[0,0,cos(theta),sin(theta),-vx*sin(theta)+vy*cos(theta),0]
    [0,0,sin(theta),-cos(theta),vx*cos(theta)+vy*sin(theta),0]
    [0,0,0,0,1,0]
    [0,0,0,0,0,1]];
Z=([v,vr,dtheta,w])';%[left,right]
R = diag([0.001,0.001, 0.001, 0.001]);
error=input_sensor_data_extant-Z;

%%
% input_sensor_data_extant=[v_input,w_input]';
% vx=state_variable_current(3);
% vy=state_variable_current(4);
% v=vx*cos(theta)+vy*sin(theta);
% dd=sqrt((state_variable_current(1)-state_variable_last(1))^2+(state_variable_current(2)-state_variable_last(2))^2);
% dtheta = state_variable_current(5)-state_variable_last(5);
% H=[[0,0,cos(theta),sin(theta),-vx*sin(theta)+vy*cos(theta),0]
%     [0,0,0,0,0,1]];
% Z=([v,w])';%[left,right]
% R = diag([0.00001, 0.00001]);
% error=input_sensor_data_extant-Z;
%%
% H_array(:,:,count)=H;
% Z=([v-w*b,v+w*b]/r)';%[left,right]
% R = diag([0.00001, 0.00001]);
% error=input_sensor_data-Z;

temp_p=H*P*H'+R;
kalman_gain=(P*H')/(temp_p);
% K_array(:,:,count)=kalman_gain;
correct_value=kalman_gain*error;
state_variable_current=state_variable_current+correct_value;
P=P-kalman_gain*H*P;
state_variable_last=state_variable_current;
time_ms=tic;
count=count+1;
% P_array(:,:,count)=P;
y = state_variable_current;

== matlab function untitled1/IMU_fusion/IMU fusion/PoseEstimationEkf ==
  data: input_sensor_data input; y output
function y = PoseEstimationEkf(input_sensor_data)
persistent state_variable_current state_variable_last P Q;
if isempty(state_variable_current)
        state_variable_current=zeros(8,1);%[xt,yt,theta_t,vxt,vyt,wt,axt,ayt]
        state_variable_last=zeros(8,1);
        Q=diag([0.1, 0.1, 0.1,0.1, 0.1, 0.1, 0.1, 0.1]);
        P=Q;
end

%%    predict
dt=0.01;
A=[[1, 0, 0, dt, 0, 0, 0, 0]
  [0, 1, 0, 0, dt, 0, 0, 0]
  [0, 0, 1, 0, 0, dt, 0, 0]
  [0, 0, 0, 1, 0, 0, dt, 0]
  [0, 0, 0, 0, 1, 0, 0, dt]
  [0, 0, 0, 0, 0, 1, 0, 0]
  [0, 0, 0, 0, 0, 0, 1, 0]
  [0, 0, 0, 0, 0, 0, 0, 1]];
state_variable_current=A*state_variable_current;
P=A*P*A'+Q;

%%    update
theta=state_variable_current(3);
theta_last=state_variable_last(3);

ax=state_variable_current(7);
ay=state_variable_current(8);

w=state_variable_current(6);
dtheta=theta-theta_last;


ax_imu=ax*cos(theta)+ay*sin(theta);
ay_imu=-ax*sin(theta)+ay*cos(theta);

%% just IMU fusion
H=[[0, 0, -ax*sin(theta)+ay*cos(theta), 0, 0, 0, cos(theta), sin(theta)]
  [0, 0, -ax*cos(theta)-ay*sin(theta), 0, 0, 0, -sin(theta), cos(theta)]
  [0, 0, 0, 0, 0, 1, 0, 0]
  [0, 0, 1, 0, 0, 0, 0, 0]];
Z=[ax_imu, ay_imu,w,dtheta]';
R = diag([0.001,0.001,0.001,0.001]);
%[ax_imu,ay_imu,w]
input_sensor_data=[input_sensor_data;input_sensor_data(3)*dt];
error=input_sensor_data-Z;
%% correct update
temp_p=H*P*H'+R;
kalman_gain=(P*H')/(temp_p);
correct_value=kalman_gain*error;
state_variable_current=state_variable_current+correct_value;
P=P-kalman_gain*H*P;
state_variable_last=state_variable_current;
y = state_variable_current;

== matlab function untitled1/OFS odm/OFS_ODM ==
  data: dx_ofs input; y output; dy_ofs input; theta input; ofs_to_robot_x input; ofs_to_robot_y input
function y = OfsOdm(dx_ofs,dy_ofs,theta,ofs_to_robot_x,ofs_to_robot_y)
persistent  current_robot_xy last_robot_xy  last_robot_theta;
if isempty(last_robot_xy)
   last_robot_xy=[0;0];
   last_robot_theta=0;
end

current_robot_theta=theta;
current_ofs_pose=[ofs_to_robot_x;ofs_to_robot_y];


rotation_matrix_last_robot_pose=[[cos(last_robot_theta),-sin(last_robot_theta)];
    [sin(last_robot_theta),cos(last_robot_theta)]];

rotation_matrix_current_robot_pose=[[cos(current_robot_theta),-sin(current_robot_theta)];
    [sin(current_robot_theta),cos(current_robot_theta)]];
dfos=[dx_ofs;dy_ofs];
current_robot_xy=rotation_matrix_last_robot_pose*(dfos+current_ofs_pose)+last_robot_xy-rotation_matrix_current_robot_pose*current_ofs_pose;
last_robot_xy=current_robot_xy;
last_robot_theta=current_robot_theta;
y = [current_robot_xy];

== matlab function untitled1/OFS fusion ==
  data: dx_ofs_sensor input; y output; dy_ofs_sensor input; theta input; vx_ofs_sensor input; vy_ofs_sensor input
function y = OFSfusion(dx_ofs_sensor,dy_ofs_sensor,theta,vx_ofs_sensor,vy_ofs_sensor)
persistent state_variable_current state_variable_last P Q counter;
if isempty(state_variable_current)
        state_variable_current=zeros(8,1);%[xt,yt,theta_t,vxt,vyt,wt,axt,ayt]
        state_variable_last=zeros(8,1);
        Q=diag([0.1, 0.1, 0.1,0.1, 0.1, 0.1, 0.1, 0.1]);
        P=Q;
        counter=0;
end

%%    predict
dt=0.01;
A=[[1, 0, 0, dt, 0, 0, 0.5*dt^2, 0]
  [0, 1, 0, 0, dt, 0, 0, 0.5*dt^2]
  [0, 0, 1, 0, 0, dt, 0, 0]
  [0, 0, 0, 1, 0, 0, dt, 0]
  [0, 0, 0, 0, 1, 0, 0, dt]
  [0, 0, 0, 0, 0, 1, 0, 0]
  [0, 0, 0, 0, 0, 0, 1, 0]
  [0, 0, 0, 0, 0, 0, 0, 1]];
state_variable_current=A*state_variable_current;
P=A*P*A'+Q;

%%    update
theta=state_variable_current(3);
theta_last=state_variable_last(3);
vx=state_variable_current(4);
vy=state_variable_current(5);
ax=state_variable_current(7);
ay=state_variable_current(8);
dx=state_variable_current(1)-state_variable_last(1);
dy=state_variable_current(2)-state_variable_last(2);
w=state_variable_current(6);
dtheta=theta-theta_last;

dd=sqrt(dx^2+dy^2);

dx_ofs=dd*cos(dtheta/2);
dy_ofs=dd*sin(dtheta/2);
%% all sensor data fusion  --not debug
H=[[cos(0.5*dtheta)*cos(theta_last+0.5*dtheta), cos(0.5*dtheta)*sin(theta_last+0.5*dtheta), -0.5*dd*sin(0.5*dtheta), 0, 0, 0, 0, 0]
   [sin(0.5*dtheta)*cos(theta_last+0.5*dtheta), sin(0.5*dtheta)*sin(theta_last+0.5*dtheta), 0.5*dd*cos(0.5*dtheta), 0, 0, 0, 0, 0]];
Z=[dx_ofs,dy_ofs]';
R = diag([0.001,0.001]);
ofs_input_sensor_data=[dx_ofs_sensor;dy_ofs_sensor];
error=ofs_input_sensor_data-Z;


%% correct update
temp_p=H*P*H'+R;
kalman_gain=(P*H')/(temp_p);
correct_value=kalman_gain*error;
state_variable_current=state_variable_current+correct_value;
P=P-kalman_gain*H*P;
state_variable_last=state_variable_current;
counter=counter+1;
y = state_variable_current;

== matlab function untitled1/OFS reader/MATLAB Function ==
  data: ofs_pose_robot input; y output; robot_pose input
function y = fcn(ofs_pose_robot,robot_pose)

persistent current_robot_xy last_robot_xy  last_robot_theta;
if isempty(last_robot_xy)
   last_robot_xy=[0;0];
   last_robot_theta=0;
end

current_robot_xy=[robot_pose(1);robot_pose(2)];
current_robot_theta=robot_pose(3);
current_ofs_pose=[ofs_pose_robot(1);ofs_pose_robot(2)];


rotation_matrix_last_robot_pose=[[cos(last_robot_theta),-sin(last_robot_theta)];
    [sin(last_robot_theta),cos(last_robot_theta)]];

rotation_matrix_current_robot_pose=[[cos(current_robot_theta),-sin(current_robot_theta)];
    [sin(current_robot_theta),cos(current_robot_theta)]];

dfos=inv(rotation_matrix_last_robot_pose)*(current_robot_xy-last_robot_xy+rotation_matrix_current_robot_pose*current_ofs_pose)-current_ofs_pose;
last_robot_xy=current_robot_xy;
last_robot_theta=current_robot_theta;
y = dfos;
